simulink model "FRAME_SIM"  (R2018b)
settings: Solver=VariableStepAuto  StartTime=0.0  StopTime=15  RelTol=1e-3
undefined symbols (not defined in the file or in its folder): serial
libraries: instrumentlib x3
settings Model: Creator=Marek  LastModifiedBy=pawwc
settings SFSimCC: SimUseLocalCustomCode=off
settings RTWCC: RTWUseLocalCustomCode=off
settings CodeAppCC: StateflowObjectComments=on

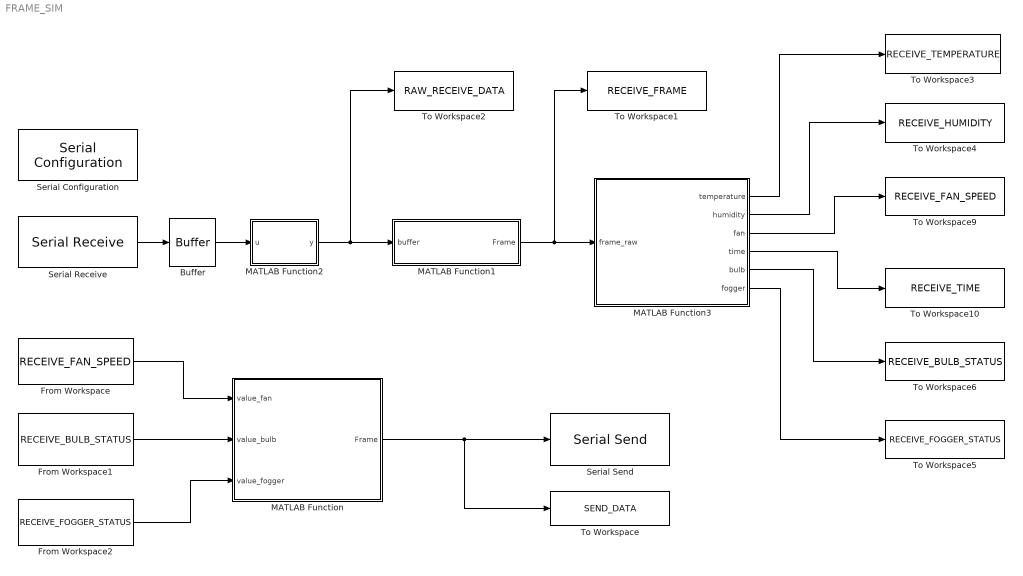
== system FRAME_SIM ==
  Buffer : Buffer  N=50  OutputFrames=off
  From Workspace : FromWorkspace  VariableName=RECEIVE_FAN_SPEED  SampleTime=0
  From Workspace1 : FromWorkspace  VariableName=RECEIVE_BULB_STATUS  SampleTime=0
  From Workspace2 : FromWorkspace  VariableName=RECEIVE_FOGGER_STATUS  SampleTime=0
  MATLAB Function : MATLAB Function  TreatAsAtomicUnit=on
  MATLAB Function1 : MATLAB Function  TreatAsAtomicUnit=on
  MATLAB Function2 : MATLAB Function  TreatAsAtomicUnit=on
  MATLAB Function3 : MATLAB Function  TreatAsAtomicUnit=on
  Serial Configuration : instrumentlib/Serial Configuration  Priority=-200000  ComPortMenu=<Please select a port...>  ComPort=COM9  ObjConstructor=serial('COM9');  BaudRate=9600  DataBits=8  Parity=none  StopBits=1  FlowControl=none  Timeout=1  ByteOrder=BigEndian
  Serial Receive : instrumentlib/Serial Receive  ComPortMenu=<Please select a port...>  ComPort=COM9  ObjConstructor=serial('COM9');  Terminator=<none>  DataSize=1  DataType=uint8  EnableBlockingMode=on  ActionDataUnavailable=Output last received value  CustomValue=0  SampleTime=0.01
  Serial Send : instrumentlib/Serial Send  ComPortMenu=<Please select a port...>  ComPort=COM9  ObjConstructor=serial('COM9');  Terminator=<none>  EnableBlockingMode=off
  To Workspace : ToWorkspace  VariableName=SEND_DATA  SampleTime=-1
  To Workspace1 : ToWorkspace  VariableName=RECEIVE_FRAME  SampleTime=-1
  To Workspace10 : ToWorkspace  VariableName=RECEIVE_TIME  SampleTime=-1
  To Workspace2 : ToWorkspace  VariableName=RAW_RECEIVE_DATA  SampleTime=-1
  To Workspace3 : ToWorkspace  VariableName=RECEIVE_TEMPERATURE  SampleTime=-1
  To Workspace4 : ToWorkspace  VariableName=RECEIVE_HUMIDITY  SampleTime=-1
  To Workspace5 : ToWorkspace  VariableName=RECEIVE_FOGGER_STATUS  SampleTime=-1
  To Workspace6 : ToWorkspace  VariableName=RECEIVE_BULB_STATUS  SampleTime=-1
  To Workspace9 : ToWorkspace  VariableName=RECEIVE_FAN_SPEED  SampleTime=-1
  wires:
  MATLAB Function/1(Frame) -> To Workspace/1, Serial Send/1
  Serial Receive/1 -> Buffer/1
  Buffer/1 -> MATLAB Function2/1(u)
  MATLAB Function1/1(Frame) -> To Workspace1/1, MATLAB Function3/1(frame_raw)
  MATLAB Function2/1(y) -> To Workspace2/1, MATLAB Function1/1(buffer)
  MATLAB Function3/1(temperature) -> To Workspace3/1
  MATLAB Function3/2(humidity) -> To Workspace4/1
  MATLAB Function3/6(fogger) -> To Workspace5/1
  MATLAB Function3/5(bulb) -> To Workspace6/1
  MATLAB Function3/4(time) -> To Workspace10/1
  MATLAB Function3/3(fan) -> To Workspace9/1
  From Workspace2/1 -> MATLAB Function/3(value_fogger)
  From Workspace1/1 -> MATLAB Function/2(value_bulb)
  From Workspace/1 -> MATLAB Function/1(value_fan)

== matlab function FRAME_SIM/MATLAB Function1 ==
  data: buffer input; Frame output

function Frame = search_frame_fcn(buffer)

buffer_size=length(buffer);
FRAME_SIZE=14;
start_code=hex2dec('40');
end_code=hex2dec('80');
Frame = zeros(1,14);

for i=1:(buffer_size-FRAME_SIZE)
   if( (buffer(i) == start_code) && (buffer(i+(FRAME_SIZE-1)) == end_code))  
       for j=1:FRAME_SIZE
           Frame(j) = buffer(i + j-1);
       end
       break
   end
end

== matlab function FRAME_SIM/MATLAB Function ==
  data: Frame output size=[1 14]; value_fan input; value_bulb input; value_fogger input
function Frame = fcn(value_fan, value_bulb, value_fogger)

start_code = hex2dec('40');

% temperature = typecast(swapbytes(single(value_temperature)), 'uint8');
% humidity = typecast(swapbytes(single(value_humidity)), 'uint8');
% time = cast(value_time,'uint8');
fan = cast(value_fan,'uint8');
bulb = cast(value_bulb,'uint8');
fogger = cast(value_fogger,'uint8');

end_code = hex2dec('80');

Frame = [end_code, fogger, bulb, fan, start_code];

== matlab function FRAME_SIM/MATLAB Function2 ==
  data: u input; y output
function y = fcn(u)

y = u;

== matlab function FRAME_SIM/MATLAB Function3 ==
  data: frame_raw input; temperature output size=1; humidity output size=1; fan output size=1; time output size=1; bulb output size=1; fogger output size=1


function [temperature, humidity, fan, time, bulb, fogger] = decompresion_fcn(frame_raw)
frame = cast(frame_raw,'uint8');
temperature=typecast(frame(2:5),'single');
humidity=typecast(frame(6:9),'single');
fan=typecast(frame(10),'uint8');
time=typecast(frame(11),'uint8');
bulb=typecast(frame(12),'uint8');
fogger=typecast(frame(13),'uint8');
end
